simulink model "sampleModel186"  (R2021b)
settings: Solver=VariableStepAuto  StartTime=0.0  StopTime=10.0  RelTol=1e-3
undefined symbols (not defined in the file or in its folder): DiscIntNeverNeededParam, Newton, Raphson
libraries: simulink x19, slpidlib x2
settings Model: Creator=user  LastModifiedBy=user

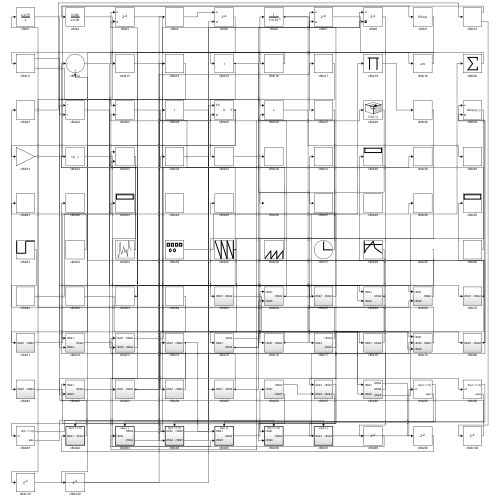
[thumbnail: Simulink's stored preview of the top-level diagram]
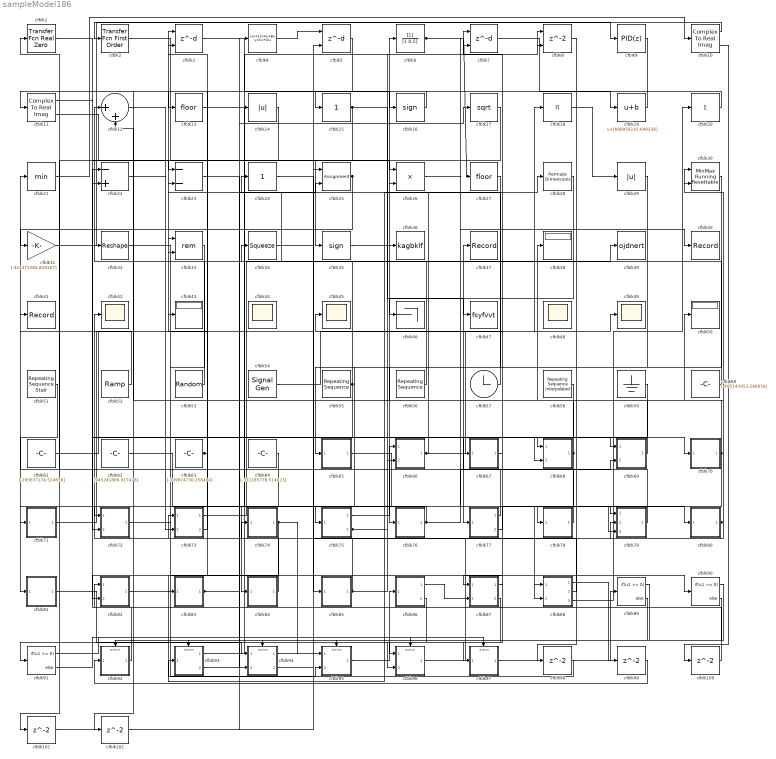
== system sampleModel186 ==
  cfblk1 : simulink/Discrete/Transfer Fcn Real Zero  ZeroZ=0.75  ICPrevInput=0.0  DoSatur=off
      settings: SourceProductBaseCode=SL
  cfblk10 : ComplexToRealImag
  cfblk{98..102} (5 alike) : Delay  SampleTime=1
  cfblk11 : ComplexToRealImag
  cfblk12 : Sum  Inputs=|++
  cfblk13 : Rounding
  cfblk14 : Abs
  cfblk15 : simulink/Math Operations/Slider Gain  gain=1  low=0  high=2
  cfblk16 : Signum
  cfblk17 : Sqrt  SaturateOnIntegerOverflow=on
  cfblk18 : Product  Inputs=*
  cfblk19 : Bias  Bias=[668959142.646336]
  cfblk2 : simulink/Discrete/Transfer Fcn First Order  PoleZ=0.95  ICPrevOutput=0.0  DoSatur=off
  cfblk20 : Sum  Inputs=+
  cfblk21 : MinMax
  cfblk22 : Sum  Inputs=-+
  cfblk23 : Sum  Inputs=--
  cfblk24 : simulink/Math Operations/Slider Gain  gain=1  low=0  high=2
  cfblk25 : Assignment  DiagnosticForDimensions=Warning  IndexOptions=Index vector (dialog)  Indices=1  OutputSizes=1
  cfblk26 : Product  Inputs=**
  cfblk27 : Rounding
  cfblk28 : PermuteDimensions
  cfblk29 : Abs
  cfblk3 : Delay  DelayLengthSource=Input port  SampleTime=1
      settings: InputPortMap=u0,p1
  cfblk30 : simulink/Math Operations/MinMax Running Resettable  Function=min  vinit=0.0
  cfblk31 : Gain  Gain=[-424473284.828187]
  cfblk32 : Reshape
  cfblk33 : Math  Operator=rem  SaturateOnIntegerOverflow=on
  cfblk34 : Squeeze
  cfblk35 : Signum
  cfblk36 : ToWorkspace  VariableName=kagbklf  SaveFormat=Timeseries  SampleTime=-1
  cfblk37 : Record  FileSettingsInternal="{\"entries\":[{\"content\":{\"excelSettings\":{\"content\":{},\"type\":\"Streamout.ExcelSettings\"}},\"type\":\"Streamout.FileSettingStorage\",\"uuid\":\"361a29f1-e2fb-4c0b-8be8-713980ecb456\"}],\"packageUris\":[\"http://schema.mathworks.com/mf0/streamout_blocks/R2020a\"],\"version\":\"1.0\"}"  SignalsInternal="{\"entries\":[{\"content\":{\"signals\":[{\"content\":{\"blockPath\":[\"sampleModel186/cfblk37\"],\"channel\":[],\"dimensions\":[1],\"domain\":\"sampleModel186/cfblk37\",\"lineColor\":\"#a2142f\",\"plots\":[1],\"port\":1,\"sid\":[\"\"],\"signalID\":6959,\"signalName\":\"cfblk77:1\"},\"type\":\"RecordBlkView.Signal\",\"uuid\":\"633224d4-002b-45fd-b44c-2713e6f3cb67\"}]},\"type\":\"RecordBlkView.InputSignals\",\"uuid\":\"d19c6e63-8a72-4a50-befe-2383d5ad5215\"}],\"packageUris\":[\"http://schema.mathworks.com/mf0/streamout_blocks/R2020a\"],\"version\":\"1.0\"}"  VisualizationBindings="{\"sparklinesplugin\":{\"info\":[{\"bindingParametersList\":[],\"subplotID\":1}]}}"
  cfblk38 : Display
  cfblk39 : ToWorkspace  VariableName=ojdnert  SaveFormat=Timeseries  SampleTime=-1
  cfblk4 : DiscreteStateSpace
  cfblk40 : Record  FileSettingsInternal="{\"entries\":[{\"content\":{\"excelSettings\":{\"content\":{},\"type\":\"Streamout.ExcelSettings\"}},\"type\":\"Streamout.FileSettingStorage\",\"uuid\":\"335357aa-7939-4387-8d3e-96902769ceac\"}],\"packageUris\":[\"http://schema.mathworks.com/mf0/streamout_blocks/R2020a\"],\"version\":\"1.0\"}"  SignalsInternal="{\"entries\":[{\"content\":{\"signals\":[{\"content\":{\"blockPath\":[\"sampleModel186/cfblk40\"],\"channel\":[],\"dimensions\":[1],\"domain\":\"sampleModel186/cfblk40\",\"lineColor\":\"#4dbeee\",\"plots\":[1],\"port\":1,\"sid\":[\"\"],\"signalID\":6955,\"signalName\":\"cfblk26\"},\"type\":\"RecordBlkView.Signal\",\"uuid\":\"b43d4440-5883-4200-968a-5c1987ee6076\"}]},\"type\":\"RecordBlkView.InputSignals\",\"uuid\":\"f55b186d-9257-4222-a712-8ac48577baf3\"}],\"packageUris\":[\"http://schema.mathworks.com/mf0/streamout_blocks/R2020a\"],\"version\":\"1.0\"}"  VisualizationBindings="{\"sparklinesplugin\":{\"info\":[{\"bindingParametersList\":[],\"subplotID\":1}]}}"
  cfblk41 : Record  FileSettingsInternal="{\"entries\":[{\"content\":{\"excelSettings\":{\"content\":{},\"type\":\"Streamout.ExcelSettings\"}},\"type\":\"Streamout.FileSettingStorage\",\"uuid\":\"56ab8f88-1f3f-40e9-89f9-4753a7ceaef6\"}],\"packageUris\":[\"http://schema.mathworks.com/mf0/streamout_blocks/R2020a\"],\"version\":\"1.0\"}"  SignalsInternal="{\"entries\":[{\"content\":{\"signals\":[{\"content\":{\"blockPath\":[\"sampleModel186/cfblk41\"],\"channel\":[],\"dimensions\":[1],\"domain\":\"sampleModel186/cfblk41\",\"lineColor\":\"#139fff\",\"plots\":[1],\"port\":1,\"sid\":[\"\"],\"signalID\":6963,\"signalName\":\"cfblk52\"},\"type\":\"RecordBlkView.Signal\",\"uuid\":\"2a08bd36-c2ee-4411-9ab5-2944906db4bc\"}]},\"type\":\"RecordBlkView.InputSignals\",\"uuid\":\"1cdacadd-d533-4878-aea6-50ff4e90bca4\"}],\"packageUris\":[\"http://schema.mathworks.com/mf0/streamout_blocks/R2020a\"],\"version\":\"1.0\"}"  VisualizationBindings="{\"sparklinesplugin\":{\"info\":[{\"bindingParametersList\":[],\"subplotID\":1}]}}"
  cfblk{42,44..45,48..49} (5 alike) : Scope
      cfblk44 settings: Floating=on
      cfblk48 settings: Floating=on
  cfblk43 : Display
  cfblk46 : Terminator
  cfblk47 : ToWorkspace  VariableName=fsyfvvt  SaveFormat=Timeseries  SampleTime=-1
  cfblk5 : Delay  DelayLengthSource=Input port  SampleTime=1
      settings: InputPortMap=u0,p1
  cfblk50 : Display
  cfblk51 : simulink/Sources/Repeating Sequence Stair  OutValues=[620580449.929200, 870089147.152765]  tsamp=-1  OutMin=[]  OutMax=[]  OutDataTypeStr=double  OutputDataTypeScalingMode=double  OutDataType=fixdt(0,8)  ConRadixGroup=Best Precision: Vector-wise  OutScaling=2^-12
  cfblk52 : simulink/Sources/Ramp  slope=[-8361.803959]  start=[45.937511]  InitialOutput=[851398.023943]
  cfblk53 : UniformRandomNumber  Minimum=[-2789928258.218382]  Maximum=[1410879306.297932]  Seed=[32986250.000000]  SampleTime=0.1
  cfblk54 : SignalGenerator  Amplitude=[294604167.686260]
  cfblk55 : simulink/Sources/Repeating Sequence  rep_seq_t=[0 2]  rep_seq_y=[231144790.500168, -400138389.187557]
  cfblk56 : simulink/Sources/Repeating Sequence  rep_seq_t=[0 2]  rep_seq_y=[-909458064.631079, -512532606.815196]
  cfblk57 : Clock
  cfblk58 : simulink/Sources/Repeating Sequence Interpolated  OutValues=[-893593142.986158, -533793627.392967, 354915419.604985, -376063202.621054, -932854939.160341]  TimeValues=[0 0.1 0.5 0.6 1].'  LookUpMeth=Use Input Above  tsamp=0.01  OutMin=[]  OutMax=[]  OutDataTypeStr=double  OutputDataTypeScalingMode=double  OutDataType=fixdt(0,8)  OutScaling=2^-10
  cfblk59 : Ground
  cfblk6 : DiscreteFilter  SampleTime=1
  cfblk60 : Constant  Value=[-695143953.286656]  SampleTime=1
  cfblk61 : Constant  Value=[-295637174.524656]  SampleTime=1
  cfblk62 : Constant  Value=[945241806.917478]  SampleTime=1
  cfblk63 : Constant  Value=[-309874730.258494]  SampleTime=1
  cfblk64 : Constant  Value=[-321185778.514623]  SampleTime=1
  cfblk65 : Subsystem
  cfblk66 : Subsystem
  cfblk67 : Subsystem
  cfblk68 : Subsystem
  cfblk69 : Subsystem
  cfblk7 : Delay  DelayLengthSource=Input port  SampleTime=1
      settings: InputPortMap=u0,p1
  cfblk70 : Subsystem
  cfblk71 : Subsystem
  cfblk72 : Subsystem
  cfblk73 : Subsystem
  cfblk74 : Subsystem
  cfblk75 : Subsystem
  cfblk76 : Subsystem
  cfblk77 : Subsystem
  cfblk78 : Subsystem
  cfblk79 : Subsystem
  cfblk8 : Delay  ShowEnablePort=on  SampleTime=1
      settings: InputPortMap=u0,e6
  cfblk80 : Subsystem
  cfblk81 : Subsystem
  cfblk82 : Subsystem
  cfblk83 : Subsystem
  cfblk84 : Subsystem
  cfblk85 : Subsystem
  cfblk86 : Subsystem
  cfblk87 : Subsystem
  cfblk88 : Subsystem
  cfblk89 : If  IfExpression=u1 >= 0  SampleTime=1
  cfblk9 : slpidlib/PID Controller  Controller=PID  Form=Parallel  TimeDomain=Discrete-time  UseExternalTs=off  SampleTime=1  IntegratorMethod=Forward Euler  FilterMethod=Forward Euler  ControllerParametersSource=internal  P=1  I=1  D=0  UseFilter=on  N=100  TunerSelectOption=Transfer Function Based (PID Tuner App)  InitialConditionSource=internal  InitialConditionForIntegrator=0  InitialConditionForFilter=0  DifferentiatorICPrevScaledInput=0  ExternalReset=none  TrackingMode=off  Kt=1  LimitOutput=off  SatLimitsSource=internal  UpperSaturationLimit=inf  LowerSaturationLimit=-inf  LinearizeAsGain=off  AntiWindupMode=none  Kb=1  POutMin=[]  POutMax=[]  IOutMin=[]  IOutMax=[]  DOutMin=[]  DOutMax=[]  NOutMin=[]  NOutMax=[]  SumOutMin=[]  SumOutMax=[]  SaturationOutMin=[]  SaturationOutMax=[]  PParamMin=[]  PParamMax=[]  IParamMin=[]  IParamMax=[]  DParamMin=[]  DParamMax=[]  NParamMin=[]  NParamMax=[]  KbParamMin=[]  KbParamMax=[]  KtParamMin=[]  KtParamMax=[]  KbOutMin=[]  KbOutMax=[]  KtOutMin=[]  KtOutMax=[]  IntegratorOutMin=[]  IntegratorOutMax=[]  FilterOutMin=[]  FilterOutMax=[]  SumI1OutMin=[]  SumI1OutMax=[]  SumI2OutMin=[]  SumI2OutMax=[]  SumI3OutMin=[]  SumI3OutMax=[]  SumI4OutMin=[]  SumI4OutMax=[]  SumDOutMin=[]  SumDOutMax=[]  DifferentiatorOutMin=[]  DifferentiatorOutMax=[]  FilterDiffOutCoefMin=[]  FilterDiffOutCoefMax=[]  ReciprocalOutMin=[]  ReciprocalOutMax=[]  SumDenOutMin=[]  SumDenOutMax=[]  SumNumOutMin=[]  SumNumOutMax=[]  DivideOutMin=[]  DivideOutMax=[]  UdiffTsProdOutMin=[]  UdiffTsProdOutMax=[]  NTsProdOutMin=[]  NTsProdOutMax=[]  UintegralTsProdOutMin=[]  UintegralTsProdOutMax=[]  UngainTsProdOutMin=[]  UngainTsProdOutMax=[]  IntegratorContinuousStateAttributes=''  IntegratorStateMustResolveToSignalObject=off  IntegratorRTWStateStorageClass=Auto  FilterContinuousStateAttributes=''  FilterStateMustResolveToSignalObject=off  FilterRTWStateStorageClass=Auto  ParallelPVariant=InternalParameters  IdealPVariant=Disabled  IVariant=InternalParameters  DVariant=InternalParameters  IntegratorVariant=Discrete  SatVariant=Disabled  AWVariant=Passthrough  PCopyVariant=Disabled  TRVariant=Disabled  FdbkBlocksVariant=Forward  IdealPFdbkVariant=Disabled  SatFdbkVariant=Disabled  DerivativeFilterVariant=ForwardEulerFilter  NVariant=InternalParameters  NCopyVariant=Disabled  FilterICVariant=InternalICsFilter  IntegratorICVariant=InternalICs  ExternalResetVariant=Disabled  TRSumVariant=Passthrough  SumFdbkVariant=Disabled  SumVariant=Sum_PID  TsampFilterVariant=InternalTs  TsampNgainVariant=Passthrough  TsampIntegralVariant=Passthrough  ExternalSaturationOutDataTypeStr=Inherit: Same as second input
  cfblk90 : If  IfExpression=u1 >= 0  SampleTime=1
  cfblk91 : If  IfExpression=u1 >= 0  SampleTime=1
  cfblk92 : Subsystem  TreatAsAtomicUnit=on
  cfblk93 : Subsystem  TreatAsAtomicUnit=on
  cfblk94 : Subsystem  TreatAsAtomicUnit=on
  cfblk95 : Subsystem  TreatAsAtomicUnit=on
  cfblk96 : Subsystem  TreatAsAtomicUnit=on
  cfblk97 : Subsystem  TreatAsAtomicUnit=on
  wires:
  cfblk93/1(cfblk2) -> cfblk8/1
  cfblk74/1(cfblk2) -> cfblk95/1(cfblk1), cfblk82/2(cfblk5)
  cfblk29/1 -> cfblk76/1(cfblk1)
  cfblk33/1 -> cfblk95/2(cfblk5)
  cfblk31/1 -> cfblk9/1
  cfblk15/1 -> cfblk35/1, cfblk47/1
  cfblk64/1 -> cfblk84/1(cfblk1)
  cfblk53/1 -> cfblk12/1
  cfblk51/1 -> cfblk81/1(cfblk1)
  cfblk82/1(cfblk2) -> cfblk28/1
  cfblk13/1 -> cfblk80/1(cfblk1)
  cfblk77/1(cfblk2) -> cfblk37/1
  cfblk6/1 -> cfblk27/1, cfblk79/3(cfblk4)
  cfblk60/1 -> cfblk32/1
  cfblk59/1 -> cfblk77/1(cfblk1)
  cfblk27/1 -> cfblk65/1(cfblk1)
  cfblk56/1 -> cfblk34/1
  cfblk21/1 -> cfblk10/1
  cfblk10/1 -> cfblk2/1
  cfblk79/1(cfblk2) -> cfblk21/1
  cfblk69/1(cfblk2) -> cfblk6/1
  cfblk25/1 -> cfblk31/1, cfblk72/1(cfblk1)
  cfblk96/1(cfblk2) -> cfblk50/1
  cfblk95/1(cfblk2) -> cfblk86/1(cfblk1)
  cfblk3/1 -> cfblk16/1
  cfblk24/1 -> cfblk85/1(cfblk1)
  cfblk83/1(cfblk2) -> cfblk17/1, cfblk25/2
  cfblk75/1(cfblk2) -> cfblk66/1(cfblk1)
  cfblk2/1 -> cfblk26/1
  cfblk70/1(cfblk2) -> cfblk87/1(cfblk1), cfblk12/2, cfblk33/2
  cfblk57/1 -> cfblk3/1
  cfblk66/1(cfblk2) -> cfblk49/1, cfblk26/2
  cfblk11/1 -> cfblk23/1
  cfblk93/2(cfblk4) -> cfblk14/1
  cfblk18/1 -> cfblk29/1
  cfblk52/1 -> cfblk41/1
  cfblk7/1 -> cfblk19/1
  cfblk77/2(cfblk5) -> cfblk45/1
  cfblk28/1 -> cfblk46/1
  cfblk55/1 -> cfblk24/1, cfblk72/2(cfblk4)
  cfblk61/1 -> cfblk23/2
  cfblk81/1(cfblk2) -> cfblk94/1(cfblk1)
  cfblk34/1 -> cfblk78/1(cfblk1)
  cfblk65/1(cfblk2) -> cfblk88/1(cfblk1)
  cfblk88/2(cfblk4) -> cfblk73/1(cfblk1)
  cfblk72/1(cfblk2) -> cfblk90/1
  cfblk85/1(cfblk2) -> cfblk66/2(cfblk5), cfblk74/1(cfblk1)
  cfblk86/1(cfblk2) -> cfblk87/2(cfblk3)
  cfblk88/3(cfblk5) -> cfblk20/1
  cfblk16/1 -> cfblk11/1
  cfblk26/1 -> cfblk40/1
  cfblk20/1 -> cfblk13/1
  cfblk19/1 -> cfblk15/1
  cfblk1/1 -> cfblk70/1(cfblk1)
  cfblk22/1 -> cfblk69/1(cfblk1)
  cfblk73/1(cfblk2) -> cfblk39/1
  cfblk4/1 -> cfblk5/1
  cfblk54/1 -> cfblk18/1
  cfblk62/1 -> cfblk88/2(cfblk3)
  cfblk12/1 -> cfblk68/1(cfblk1)
  cfblk94/1(cfblk2) -> cfblk8/2
  cfblk11/2 -> cfblk73/2(cfblk3)
  cfblk86/2(cfblk5) -> cfblk91/1
  cfblk30/1 -> cfblk75/1(cfblk1)
  cfblk32/1 -> cfblk67/1(cfblk1)
  cfblk63/1 -> cfblk3/2, cfblk33/1
  cfblk68/1(cfblk2) -> cfblk38/1, cfblk97/1(cfblk1)
  cfblk97/1(cfblk2) -> cfblk89/1
  cfblk73/2(cfblk4) -> cfblk43/1
  cfblk84/1(cfblk2) -> cfblk42/1
  cfblk80/1(cfblk2) -> cfblk30/1, cfblk30/2
  cfblk87/1(cfblk2) -> cfblk96/1(cfblk1)
  cfblk87/2(cfblk4) -> cfblk96/2(cfblk4)
  cfblk35/1 -> cfblk36/1
  cfblk67/1(cfblk2) -> cfblk7/1
  cfblk14/1 -> cfblk22/2
  cfblk75/2(cfblk5) -> cfblk79/1(cfblk1), cfblk7/2
  cfblk71/1(cfblk2) -> cfblk25/1
  cfblk92/1(cfblk2) -> cfblk82/1(cfblk1)
  cfblk23/1 -> cfblk68/2(cfblk4)
  cfblk78/1(cfblk2) -> cfblk1/1
  cfblk58/1 -> cfblk94/2(cfblk4)
  cfblk76/1(cfblk2) -> cfblk69/2(cfblk4), cfblk71/1(cfblk1)
  cfblk94/2(cfblk5) -> cfblk79/2(cfblk3)
  cfblk5/1 -> cfblk83/1(cfblk1)
  cfblk89/1 -> cfblk92/Action
  cfblk89/2 -> cfblk93/Action
  cfblk90/1 -> cfblk94/Action
  cfblk90/2 -> cfblk95/Action
  cfblk91/1 -> cfblk96/Action
  cfblk91/2 -> cfblk97/Action
  cfblk8/1 -> cfblk98/1
  cfblk98/1 -> cfblk93/1(cfblk1)
  cfblk88/1(cfblk2) -> cfblk99/1
  cfblk99/1 -> cfblk92/1(cfblk1)
  cfblk10/2 -> cfblk100/1
  cfblk100/1 -> cfblk22/1
  cfblk17/1 -> cfblk101/1
  cfblk101/1 -> cfblk5/2
  cfblk9/1 -> cfblk102/1
  cfblk102/1 -> cfblk4/1

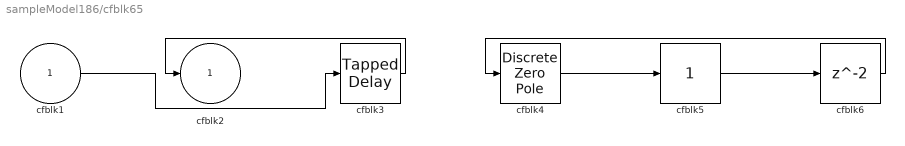
== system sampleModel186/cfblk65 ==
  cfblk1 : Inport
  cfblk3 : simulink/Discrete/Tapped Delay  vinit=0.0  samptime=-1  NumDelays=1  DelayOrder=Oldest  includeCurrent=off
  cfblk4 : DiscreteZeroPole  Poles=[0 0.5]  Gain=1
  cfblk5 : simulink/Math Operations/Slider Gain  gain=1  low=0  high=2
  cfblk6 : Delay  SampleTime=1
  cfblk2 : Outport
  wires:
  cfblk3/1 -> cfblk2/1
  cfblk1/1 -> cfblk3/1
  cfblk4/1 -> cfblk5/1
  cfblk5/1 -> cfblk6/1
  cfblk6/1 -> cfblk4/1

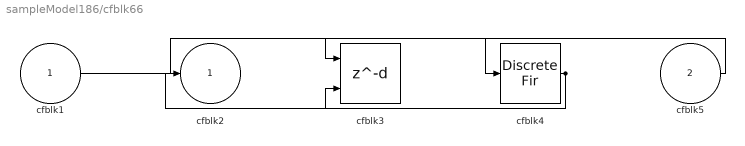
== system sampleModel186/cfblk66 ==
  cfblk1 : Inport
  cfblk5 : Inport  Port=2
  cfblk3 : Delay  DelayLengthSource=Input port  SampleTime=1
      settings: InputPortMap=u0,p1
  cfblk4 : DiscreteFir  SampleTime=1
  cfblk2 : Outport
  wires:
  cfblk1/1 -> cfblk4/1
  cfblk4/1 -> cfblk2/1, cfblk3/2
  cfblk5/1 -> cfblk3/1

== system sampleModel186/cfblk67 ==
  cfblk1 : Inport
  cfblk3 : simulink/Discrete/Tapped Delay  vinit=0.0  samptime=-1  NumDelays=1  DelayOrder=Oldest  includeCurrent=off
  cfblk4 : Rounding
  cfblk2 : Outport
  wires:
  cfblk1/1 -> cfblk4/1
  cfblk3/1 -> cfblk2/1
  cfblk4/1 -> cfblk3/1

== system sampleModel186/cfblk68 ==
  cfblk1 : Inport
  cfblk4 : Inport  Port=2
  cfblk3 : Constant  Value=[610913856.524991]  SampleTime=1
  cfblk2 : Outport
  wires:
  cfblk1/1 -> cfblk2/1

== system sampleModel186/cfblk69 ==
  cfblk1 : Inport
  cfblk4 : Inport  Port=2
  cfblk3 : Abs
  cfblk2 : Outport
  wires:
  cfblk1/1 -> cfblk3/1
  cfblk3/1 -> cfblk2/1

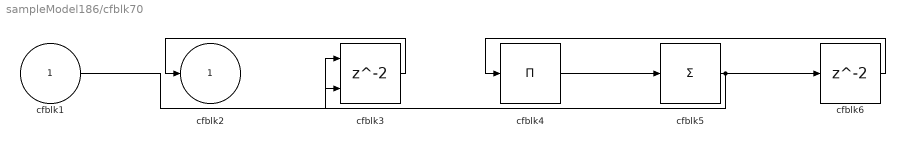
== system sampleModel186/cfblk70 ==
  cfblk1 : Inport
  cfblk3 : Delay  ShowEnablePort=on  SampleTime=1
      settings: InputPortMap=u0,e6
  cfblk4 : Product  Inputs=*
  cfblk5 : Sum  Inputs=+
  cfblk6 : Delay  SampleTime=1
  cfblk2 : Outport
  wires:
  cfblk3/1 -> cfblk2/1
  cfblk5/1 -> cfblk3/1, cfblk6/1
  cfblk4/1 -> cfblk5/1
  cfblk1/1 -> cfblk3/2
  cfblk6/1 -> cfblk4/1

== system sampleModel186/cfblk71 ==
  cfblk1 : Inport
  cfblk3 : Product  Inputs=*
  cfblk2 : Outport
  wires:
  cfblk1/1 -> cfblk2/1, cfblk3/1

== system sampleModel186/cfblk72 ==
  cfblk1 : Inport
  cfblk4 : Inport  Port=2
  cfblk3 : DiscreteIntegrator  ICPrevOutput=DiscIntNeverNeededParam  ICPrevScaledInput=DiscIntNeverNeededParam
  cfblk2 : Outport
  wires:
  cfblk1/1 -> cfblk3/1
  cfblk4/1 -> cfblk2/1

== system sampleModel186/cfblk73 ==
  cfblk1 : Inport
  cfblk3 : Inport  Port=2
  cfblk2 : Outport
  cfblk4 : Outport  Port=2
  wires:
  cfblk1/1 -> cfblk4/1
  cfblk3/1 -> cfblk2/1

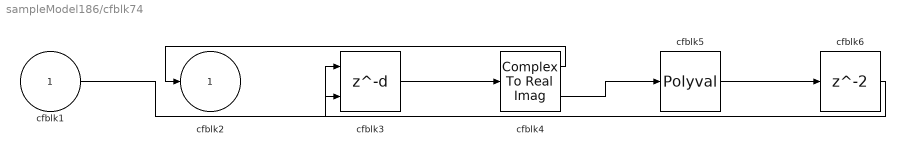
== system sampleModel186/cfblk74 ==
  cfblk1 : Inport
  cfblk3 : Delay  DelayLengthSource=Input port  SampleTime=1
      settings: InputPortMap=u0,p1
  cfblk4 : ComplexToRealImag
  cfblk5 : Polyval  Coefs=[ +2.081618890e-019, -1.441693666e-014, +4.719686976e-010, -8.536869453e-006, +1.621573104e-001, -8.087801117e+001 ]
  cfblk6 : Delay  SampleTime=1
  cfblk2 : Outport
  wires:
  cfblk4/1 -> cfblk2/1
  cfblk1/1 -> cfblk3/1
  cfblk3/1 -> cfblk4/1
  cfblk4/2 -> cfblk5/1
  cfblk5/1 -> cfblk6/1
  cfblk6/1 -> cfblk3/2

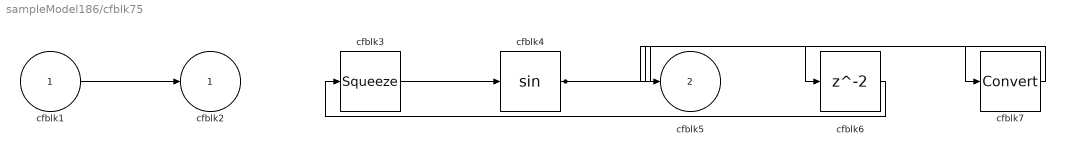
== system sampleModel186/cfblk75 ==
  cfblk1 : Inport
  cfblk3 : Squeeze
  cfblk4 : Trigonometry
  cfblk6 : Delay  SampleTime=1
  cfblk7 : DataTypeConversion
  cfblk2 : Outport
  cfblk5 : Outport  Port=2
  wires:
  cfblk1/1 -> cfblk2/1
  cfblk3/1 -> cfblk4/1
  cfblk4/1 -> cfblk6/1, cfblk7/1
  cfblk6/1 -> cfblk3/1
  cfblk7/1 -> cfblk5/1

== system sampleModel186/cfblk76 ==
  cfblk1 : Inport
  cfblk3 : DiscreteZeroPole  Poles=[0 0.5]  Gain=1
  cfblk4 : Constant  Value=[-857859279.918124]  SampleTime=1
  cfblk2 : Outport
  wires:
  cfblk1/1 -> cfblk2/1
  cfblk4/1 -> cfblk3/1

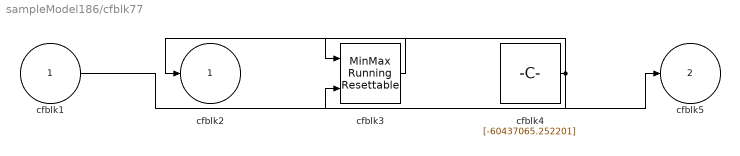
== system sampleModel186/cfblk77 ==
  cfblk1 : Inport
  cfblk3 : simulink/Math Operations/MinMax Running Resettable  Function=min  vinit=0.0
  cfblk4 : Constant  Value=[-60437065.252201]  SampleTime=1
  cfblk2 : Outport
  cfblk5 : Outport  Port=2
  wires:
  cfblk3/1 -> cfblk2/1
  cfblk1/1 -> cfblk5/1
  cfblk4/1 -> cfblk3/1, cfblk3/2

== system sampleModel186/cfblk78 ==
  cfblk1 : Inport
  cfblk3 : Product
  cfblk2 : Outport
  wires:
  cfblk1/1 -> cfblk3/1, cfblk3/2
  cfblk3/1 -> cfblk2/1

== system sampleModel186/cfblk79 ==
  cfblk1 : Inport
  cfblk3 : Inport  Port=2
  cfblk4 : Inport  Port=3
  cfblk2 : Outport
  wires:
  cfblk3/1 -> cfblk2/1

== system sampleModel186/cfblk80 ==
  cfblk1 : Inport
  cfblk3 : Sin  TimeSource=Use external signal  SampleTime=0
  cfblk4 : ComplexToMagnitudeAngle
  cfblk2 : Outport
  wires:
  cfblk3/1 -> cfblk4/1
  cfblk1/1 -> cfblk3/1
  cfblk4/1 -> cfblk2/1

== system sampleModel186/cfblk81 ==
  cfblk1 : Inport
  cfblk3 : simulink/Math Operations/Slider Gain  gain=1  low=0  high=2
  cfblk4 : Signum
  cfblk5 : Delay  SampleTime=1
  cfblk2 : Outport
  wires:
  cfblk1/1 -> cfblk2/1
  cfblk3/1 -> cfblk4/1
  cfblk4/1 -> cfblk5/1
  cfblk5/1 -> cfblk3/1

== system sampleModel186/cfblk82 ==
  cfblk1 : Inport
  cfblk5 : Inport  Port=2
  cfblk3 : slpidlib/PID Controller  Controller=PID  Form=Parallel  TimeDomain=Discrete-time  UseExternalTs=off  SampleTime=1  IntegratorMethod=Forward Euler  FilterMethod=Forward Euler  ControllerParametersSource=internal  P=1  I=1  D=0  UseFilter=on  N=100  TunerSelectOption=Transfer Function Based (PID Tuner App)  InitialConditionSource=internal  InitialConditionForIntegrator=0  InitialConditionForFilter=0  DifferentiatorICPrevScaledInput=0  ExternalReset=none  TrackingMode=off  Kt=1  LimitOutput=off  SatLimitsSource=internal  UpperSaturationLimit=inf  LowerSaturationLimit=-inf  LinearizeAsGain=off  AntiWindupMode=none  Kb=1  POutMin=[]  POutMax=[]  IOutMin=[]  IOutMax=[]  DOutMin=[]  DOutMax=[]  NOutMin=[]  NOutMax=[]  SumOutMin=[]  SumOutMax=[]  SaturationOutMin=[]  SaturationOutMax=[]  PParamMin=[]  PParamMax=[]  IParamMin=[]  IParamMax=[]  DParamMin=[]  DParamMax=[]  NParamMin=[]  NParamMax=[]  KbParamMin=[]  KbParamMax=[]  KtParamMin=[]  KtParamMax=[]  KbOutMin=[]  KbOutMax=[]  KtOutMin=[]  KtOutMax=[]  IntegratorOutMin=[]  IntegratorOutMax=[]  FilterOutMin=[]  FilterOutMax=[]  SumI1OutMin=[]  SumI1OutMax=[]  SumI2OutMin=[]  SumI2OutMax=[]  SumI3OutMin=[]  SumI3OutMax=[]  SumI4OutMin=[]  SumI4OutMax=[]  SumDOutMin=[]  SumDOutMax=[]  DifferentiatorOutMin=[]  DifferentiatorOutMax=[]  FilterDiffOutCoefMin=[]  FilterDiffOutCoefMax=[]  ReciprocalOutMin=[]  ReciprocalOutMax=[]  SumDenOutMin=[]  SumDenOutMax=[]  SumNumOutMin=[]  SumNumOutMax=[]  DivideOutMin=[]  DivideOutMax=[]  UdiffTsProdOutMin=[]  UdiffTsProdOutMax=[]  NTsProdOutMin=[]  NTsProdOutMax=[]  UintegralTsProdOutMin=[]  UintegralTsProdOutMax=[]  UngainTsProdOutMin=[]  UngainTsProdOutMax=[]  IntegratorContinuousStateAttributes=''  IntegratorStateMustResolveToSignalObject=off  IntegratorRTWStateStorageClass=Auto  FilterContinuousStateAttributes=''  FilterStateMustResolveToSignalObject=off  FilterRTWStateStorageClass=Auto  ParallelPVariant=InternalParameters  IdealPVariant=Disabled  IVariant=InternalParameters  DVariant=InternalParameters  IntegratorVariant=Discrete  SatVariant=Disabled  AWVariant=Passthrough  PCopyVariant=Disabled  TRVariant=Disabled  FdbkBlocksVariant=Forward  IdealPFdbkVariant=Disabled  SatFdbkVariant=Disabled  DerivativeFilterVariant=ForwardEulerFilter  NVariant=InternalParameters  NCopyVariant=Disabled  FilterICVariant=InternalICsFilter  IntegratorICVariant=InternalICs  ExternalResetVariant=Disabled  TRSumVariant=Passthrough  SumFdbkVariant=Disabled  SumVariant=Sum_PID  TsampFilterVariant=InternalTs  TsampNgainVariant=Passthrough  TsampIntegralVariant=Passthrough  ExternalSaturationOutDataTypeStr=Inherit: Same as second input
  cfblk4 : Sum  Inputs=+-
  cfblk2 : Outport
  wires:
  cfblk5/1 -> cfblk3/1
  cfblk1/1 -> cfblk4/1
  cfblk3/1 -> cfblk4/2
  cfblk4/1 -> cfblk2/1

== system sampleModel186/cfblk83 ==
  cfblk1 : Inport
  cfblk3 : Product
  cfblk4 : ComplexToRealImag
  cfblk2 : Outport
  wires:
  cfblk1/1 -> cfblk4/1
  cfblk4/1 -> cfblk3/1
  cfblk4/2 -> cfblk3/2
  cfblk3/1 -> cfblk2/1

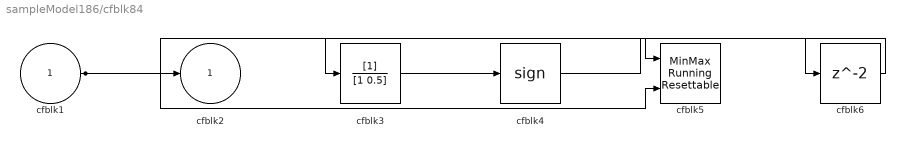
== system sampleModel186/cfblk84 ==
  cfblk1 : Inport
  cfblk3 : DiscreteFilter  SampleTime=1
  cfblk4 : Signum
  cfblk5 : simulink/Math Operations/MinMax Running Resettable  Function=min  vinit=0.0
  cfblk6 : Delay  SampleTime=1
  cfblk2 : Outport
  wires:
  cfblk3/1 -> cfblk4/1
  cfblk1/1 -> cfblk2/1, cfblk5/1, cfblk5/2
  cfblk4/1 -> cfblk6/1
  cfblk6/1 -> cfblk3/1

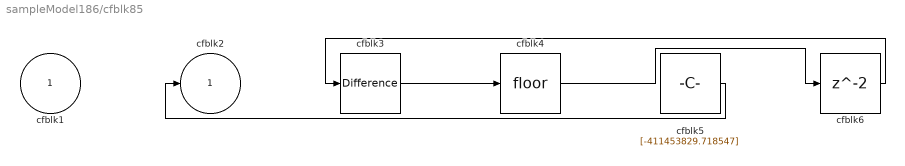
== system sampleModel186/cfblk85 ==
  cfblk1 : Inport
  cfblk3 : simulink/Discrete/Difference  ICPrevInput=0.0  OutMin=[]  OutMax=[]  OutDataTypeStr=Inherit: Inherit via back propagation  OutDataType=fixdt(1, 16)  OutScaling=2^-10  DoSatur=off
  cfblk4 : Rounding
  cfblk5 : Constant  Value=[-411453829.718547]  SampleTime=1
  cfblk6 : Delay  SampleTime=1
  cfblk2 : Outport
  wires:
  cfblk3/1 -> cfblk4/1
  cfblk5/1 -> cfblk2/1
  cfblk4/1 -> cfblk6/1
  cfblk6/1 -> cfblk3/1

== system sampleModel186/cfblk86 ==
  cfblk1 : Inport
  cfblk3 : simulink/Discrete/Difference  ICPrevInput=0.0  OutMin=[]  OutMax=[]  OutDataTypeStr=Inherit: Inherit via back propagation  OutDataType=fixdt(1, 16)  OutScaling=2^-10  DoSatur=off
  cfblk4 : Sin  TimeSource=Use external signal  SampleTime=0
  cfblk2 : Outport
  cfblk5 : Outport  Port=2
  wires:
  cfblk1/1 -> cfblk4/1
  cfblk4/1 -> cfblk2/1, cfblk3/1
  cfblk3/1 -> cfblk5/1

== system sampleModel186/cfblk87 ==
  cfblk1 : Inport
  cfblk3 : Inport  Port=2
  cfblk2 : Outport
  cfblk4 : Outport  Port=2
  wires:
  cfblk3/1 -> cfblk4/1
  cfblk1/1 -> cfblk2/1

== system sampleModel186/cfblk88 ==
  cfblk1 : Inport
  cfblk3 : Inport  Port=2
  cfblk2 : Outport
  cfblk4 : Outport  Port=2
  cfblk5 : Outport  Port=3
  wires:
  cfblk1/1 -> cfblk2/1, cfblk4/1
  cfblk3/1 -> cfblk5/1

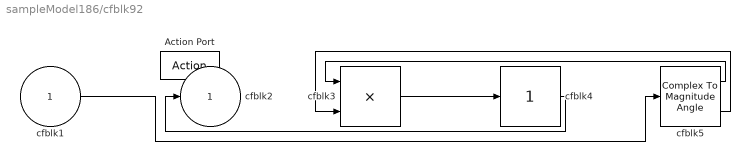
== system sampleModel186/cfblk92 ==
  cfblk1 : Inport
  Action Port : ActionPort  ActionPortLabel=if(u1 >= 0)
  cfblk3 : Product
  cfblk4 : simulink/Math Operations/Slider Gain  gain=1  low=0  high=2
  cfblk5 : ComplexToMagnitudeAngle
  cfblk2 : Outport
  wires:
  cfblk4/1 -> cfblk2/1
  cfblk3/1 -> cfblk4/1
  cfblk1/1 -> cfblk5/1
  cfblk5/1 -> cfblk3/1
  cfblk5/2 -> cfblk3/2

== system sampleModel186/cfblk93 ==
  cfblk1 : Inport
  Action Port : ActionPort  ActionPortLabel=else
  cfblk3 : DiscreteZeroPole  Poles=[0 0.5]  Gain=1  SampleTime=-1
  cfblk2 : Outport
  cfblk4 : Outport  Port=2
  wires:
  cfblk3/1 -> cfblk2/1
  cfblk1/1 -> cfblk3/1, cfblk4/1

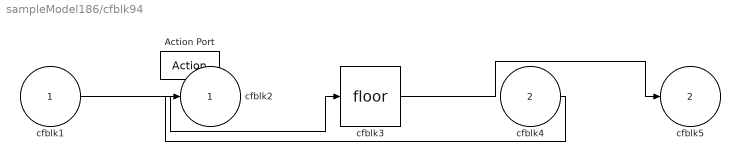
== system sampleModel186/cfblk94 ==
  cfblk1 : Inport
  cfblk4 : Inport  Port=2
  Action Port : ActionPort  ActionPortLabel=if(u1 >= 0)
  cfblk3 : Rounding
  cfblk2 : Outport
  cfblk5 : Outport  Port=2
  wires:
  cfblk3/1 -> cfblk5/1
  cfblk1/1 -> cfblk3/1
  cfblk4/1 -> cfblk2/1

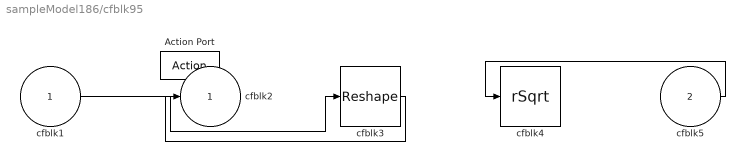
== system sampleModel186/cfblk95 ==
  cfblk1 : Inport
  cfblk5 : Inport  Port=2
  Action Port : ActionPort  ActionPortLabel=else
  cfblk3 : Reshape
  cfblk4 : Sqrt  Operator=rSqrt  AlgorithmType=Newton-Raphson  SaturateOnIntegerOverflow=on
  cfblk2 : Outport
  wires:
  cfblk5/1 -> cfblk4/1
  cfblk1/1 -> cfblk3/1
  cfblk3/1 -> cfblk2/1

== system sampleModel186/cfblk96 ==
  cfblk1 : Inport
  cfblk4 : Inport  Port=2
  Action Port : ActionPort  ActionPortLabel=if(u1 >= 0)
  cfblk3 : UnaryMinus
  cfblk2 : Outport
  wires:
  cfblk1/1 -> cfblk3/1
  cfblk4/1 -> cfblk2/1

== system sampleModel186/cfblk97 ==
  cfblk1 : Inport
  Action Port : ActionPort  ActionPortLabel=else
  cfblk3 : Product
  cfblk4 : ComplexToMagnitudeAngle
  cfblk2 : Outport
  wires:
  cfblk3/1 -> cfblk2/1
  cfblk4/1 -> cfblk3/1
  cfblk1/1 -> cfblk4/1
  cfblk4/2 -> cfblk3/2
